simulink model "fig101a"  (Simulink 3.00)
settings: Solver=ode45  StartTime=0.0  StopTime=10  RelTol=1e-3
settings Model: LimitMaxRows=on  MaxRows=50000

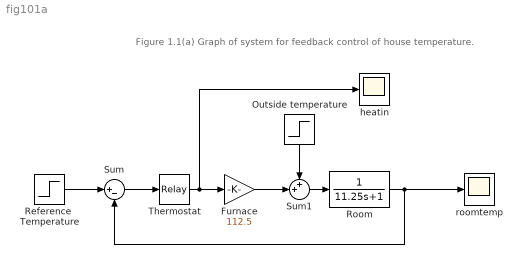
== system fig101a ==
  note: Figure 1.1(a) Graph of system for feedback control of house temperature.
  " Furnace" : Gain  Gain=112.5  SaturateOnIntegerOverflow=off
  " Outside temperature" : Step  Orientation=down  Time=0  Before=0  After=5  SampleTime=0.01
  " Reference  Temperature" : Step  Time=6  Before=10  After=20  SampleTime=0.01
  " Room" : TransferFcn  Numerator=[1]  Denominator=[11.25 1]
  " Thermostat" : Relay  OnSwitchValue=.5  OffSwitchValue=-.5  OnOutputValue=1.  OffOutputValue=0
  Sum : Sum  Inputs=|+-  SaturateOnIntegerOverflow=on
  Sum1 : Sum  Inputs=++|  SaturateOnIntegerOverflow=on
  heatin : Scope
      settings: TimeRange=auto  YMin=0  YMax=2  SaveName=heatin  DataFormat=Matrix  MaxRows=50000
  roomtemp : Scope
      settings: TimeRange=auto  YMin=-2  YMax=2  SaveName=roomtemp  DataFormat=Matrix  LimitMaxRows=off
  wires:
  " Outside temperature"/1 -> Sum1/1
  " Reference  Temperature"/1 -> Sum/1
  Sum1/1 -> " Room"/1
  " Furnace"/1 -> Sum1/2
  " Room"/1 -> Sum/2, roomtemp/1
  Sum/1 -> " Thermostat"/1
  " Thermostat"/1 -> " Furnace"/1, heatin/1
